simulink model "Modelisation_6_Validation_de_lineairisation_A_B_C"  (R2015a)
settings: Solver=ode45  StartTime=0.0  StopTime=0.2  MaxStep=0.0001  RelTol=1e-3
(part 1 of 2)
settings Model: Creator=user  LastModifiedBy=user

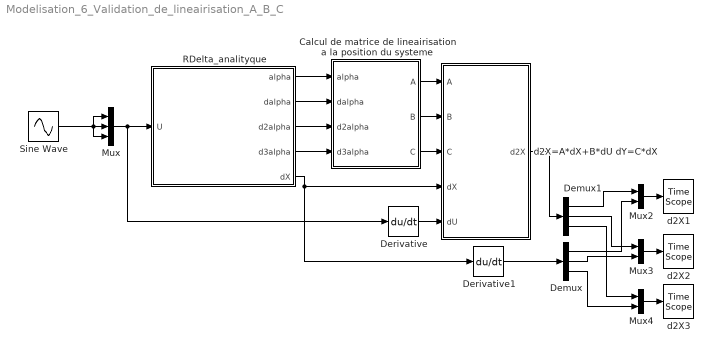
== system Modelisation_6_Validation_de_lineairisation_A_B_C ==
  Calcul de matrice de lineairisation a la position du systeme : Subsystem
  Demux : Demux  Outputs=3
  Demux1 : Demux  Outputs=3
  Derivative : Derivative
  Derivative1 : Derivative
  Mux : Mux  Inputs=3
  Mux2 : Mux  Inputs=2
  Mux3 : Mux  Inputs=2
  Mux4 : Mux  Inputs=2
  RDelta_analityque : Subsystem
      mask Display:
      | image(imread('DeltaImage2.PNG'))
      | port_label('input',1,'U')
      | port_label('output',1,'alpha')
      | port_label('output',2,'dalpha')
      | port_label('output',3,'d2alpha')
      | port_label('output',4,'d3alpha')
      | port_label('output',5,'dX')
  Sine Wave : Sin  Amplitude=0.5  SampleTime=0
  d2X1 : TimeScope  DefaultConfigurationName=spbscopes.TimeScopeBlockCfg
  d2X2 : TimeScope  DefaultConfigurationName=spbscopes.TimeScopeBlockCfg
  d2X3 : TimeScope  DefaultConfigurationName=spbscopes.TimeScopeBlockCfg
  d2X=A*dX+B*dU dY=C*dX : Subsystem
  wires:
  Calcul de matrice de lineairisation a la position du systeme/1(A) -> d2X=A*dX+B*dU dY=C*dX/1(A)
  Calcul de matrice de lineairisation a la position du systeme/2(B) -> d2X=A*dX+B*dU dY=C*dX/2(B)
  Calcul de matrice de lineairisation a la position du systeme/3(C) -> d2X=A*dX+B*dU dY=C*dX/3(C)
  RDelta_analityque/1(alpha) -> Calcul de matrice de lineairisation a la position du systeme/1(alpha)
  RDelta_analityque/2(dalpha) -> Calcul de matrice de lineairisation a la position du systeme/2(dalpha)
  RDelta_analityque/4(d3alpha) -> Calcul de matrice de lineairisation a la position du systeme/4(d3alpha)
  RDelta_analityque/3(d2alpha) -> Calcul de matrice de lineairisation a la position du systeme/3(d2alpha)
  RDelta_analityque/5(dX) -> d2X=A*dX+B*dU dY=C*dX/4(dX), Derivative1/1
  Derivative/1 -> d2X=A*dX+B*dU dY=C*dX/5(dU)
  Mux2/1 -> d2X1/1
  d2X=A*dX+B*dU dY=C*dX/1(d2X) -> Demux1/1
  Derivative1/1 -> Demux/1
  Demux1/1 -> Mux2/1
  Demux/1 -> Mux2/2
  Mux3/1 -> d2X2/1
  Demux1/2 -> Mux3/1
  Demux/2 -> Mux3/2
  Mux4/1 -> d2X3/1
  Demux1/3 -> Mux4/1
  Demux/3 -> Mux4/2
  Mux/1 -> Derivative/1, RDelta_analityque/1(U)
  Sine Wave/1 -> Mux/3, Mux/1, Mux/2

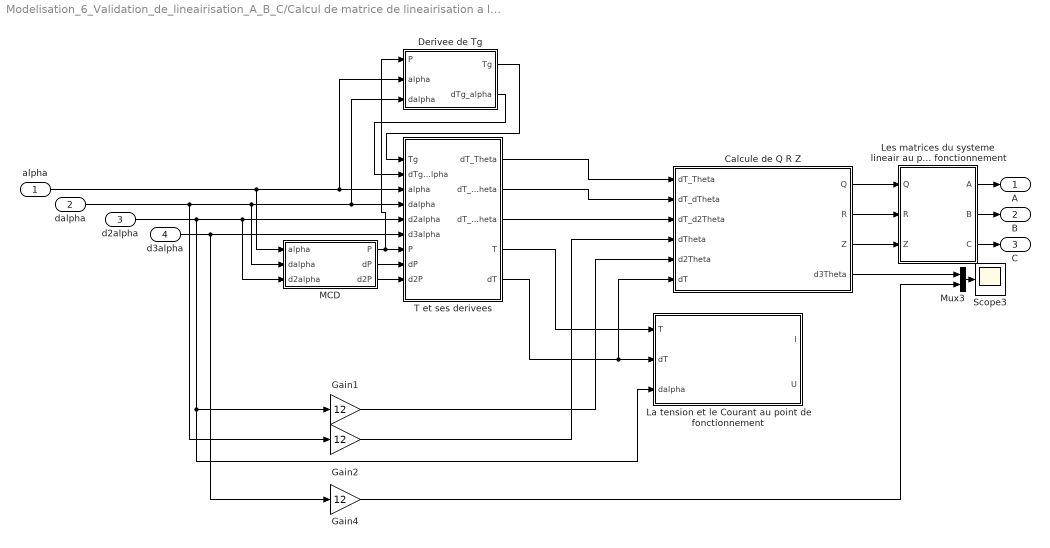
== system Modelisation_6_Validation_de_lineairisation_A_B_C/Calcul de matrice de lineairisation a la position du systeme ==
  alpha : Inport
  dalpha : Inport  Port=2
  d2alpha : Inport  Port=3
  d3alpha : Inport  Port=4
  "Calcule de Q R Z " : MATLAB Function  TreatAsAtomicUnit=on
  Derivee de Tg : Subsystem
  Gain1 : Gain  Gain=12
  Gain2 : Gain  Gain=12
  Gain4 : Gain  Gain=12
  La tension et le Courant au point de fonctionnement : MATLAB Function  TreatAsAtomicUnit=on
  Les matrices du systeme lineair au point de fonctionnement : MATLAB Function  TreatAsAtomicUnit=on
  MCD : MATLAB Function  TreatAsAtomicUnit=on
  Mux3 : Mux  Inputs=2
  Scope3 : Scope
      settings: TimeRange=2.077341948455237  YMin=-0.45  YMax=0.5
  T et ses derivees : Subsystem
  A : Outport
  B : Outport  Port=2
  C : Outport  Port=3
  wires:
  Les matrices du systeme lineair au point de fonctionnement/2(B) -> B/1
  Les matrices du systeme lineair au point de fonctionnement/3(C) -> C/1
  "Calcule de Q R Z "/1(Q) -> Les matrices du systeme lineair au point de fonctionnement/1(Q)
  "Calcule de Q R Z "/2(R) -> Les matrices du systeme lineair au point de fonctionnement/2(R)
  "Calcule de Q R Z "/3(Z) -> Les matrices du systeme lineair au point de fonctionnement/3(Z)
  Les matrices du systeme lineair au point de fonctionnement/1(A) -> A/1
  Gain4/1 -> Mux3/2
  "Calcule de Q R Z "/4(d3Theta) -> Mux3/1
  Mux3/1 -> Scope3/1
  Gain1/1 -> "Calcule de Q R Z "/5(d2Theta)
  Gain2/1 -> "Calcule de Q R Z "/4(dTheta)
  T et ses derivees/4(T) -> La tension et le Courant au point de fonctionnement/1(T)
  d3alpha/1 -> T et ses derivees/6(d3alpha), Gain4/1
  Derivee de Tg/1(Tg) -> T et ses derivees/1(Tg)
  Derivee de Tg/2(dTg_alpha) -> T et ses derivees/2(dTg_alpha)
  T et ses derivees/5(dT) -> La tension et le Courant au point de fonctionnement/2(dT), "Calcule de Q R Z "/6(dT)
  T et ses derivees/3(dT_d2Theta) -> "Calcule de Q R Z "/3(dT_d2Theta)
  T et ses derivees/2(dT_dTheta) -> "Calcule de Q R Z "/2(dT_dTheta)
  T et ses derivees/1(dT_Theta) -> "Calcule de Q R Z "/1(dT_Theta)
  d2alpha/1 -> MCD/3(d2alpha), T et ses derivees/5(d2alpha), La tension et le Courant au point de fonctionnement/3(dalpha), Gain1/1
  dalpha/1 -> MCD/2(dalpha), Derivee de Tg/3(dalpha), T et ses derivees/4(dalpha), Gain2/1
  alpha/1 -> MCD/1(alpha), T et ses derivees/3(alpha), Derivee de Tg/2(alpha)
  MCD/3(d2P) -> T et ses derivees/9(d2P)
  MCD/2(dP) -> T et ses derivees/8(dP)
  MCD/1(P) -> Derivee de Tg/1(P), T et ses derivees/7(P)

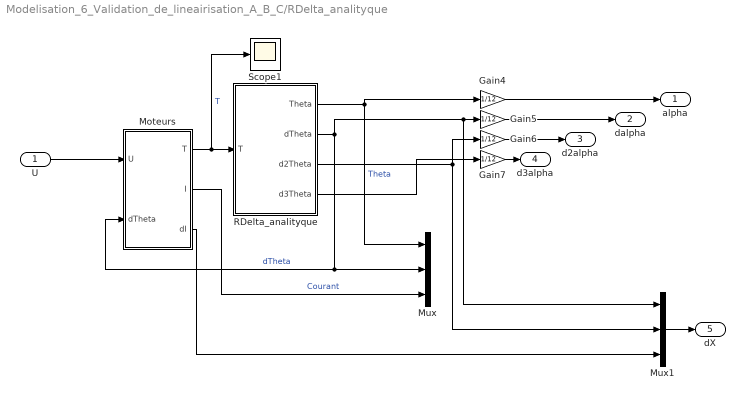
== system Modelisation_6_Validation_de_lineairisation_A_B_C/RDelta_analityque ==
  U : Inport
  Gain{4..7} (4 alike) : Gain  Gain=1/12
  Moteurs : Subsystem
  Mux : Mux  Inputs=3
  Mux1 : Mux  Inputs=3
  RDelta_analityque : Subsystem
  Scope1 : Scope
      settings: YMin=-0.013  YMax=-0.0095  SaveName=ScopeData3
  alpha : Outport
  dalpha : Outport  Port=2
  d2alpha : Outport  Port=3
  d3alpha : Outport  Port=4
  dX : Outport  Port=5
  wires:
  Moteurs/2(I) -> Mux/3  "Courant"
  U/1 -> Moteurs/1(U)
  RDelta_analityque/1(Theta) -> Mux/1, Gain4/1  "Theta"
  RDelta_analityque/2(dTheta) -> Moteurs/2(dTheta), Mux/2, Mux1/1, Gain5/1  "dTheta"
  Moteurs/1(T) -> Scope1/1, RDelta_analityque/1(T)  "T"
  RDelta_analityque/3(d2Theta) -> Mux1/2, Gain6/1
  RDelta_analityque/4(d3Theta) -> Gain7/1
  Mux1/1 -> dX/1
  Moteurs/3(dI) -> Mux1/3
  Gain4/1 -> alpha/1
  Gain5/1 -> dalpha/1
  Gain6/1 -> d2alpha/1
  Gain7/1 -> d3alpha/1

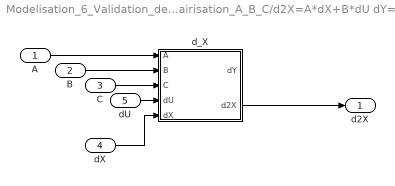
== system Modelisation_6_Validation_de_lineairisation_A_B_C/d2X=A*dX+B*dU dY=C*dX ==
  A : Inport
  B : Inport  Port=2
  C : Inport  Port=3
  dX : Inport  Port=4
  dU : Inport  Port=5
  d_X : MATLAB Function  TreatAsAtomicUnit=on
  d2X : Outport
  wires:
  B/1 -> d_X/2(B)
  C/1 -> d_X/3(C)
  A/1 -> d_X/1(A)
  dU/1 -> d_X/4(dU)
  dX/1 -> d_X/5(dX)
  d_X/2(d2X) -> d2X/1

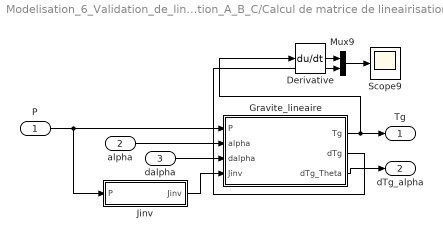
== system Modelisation_6_Validation_de_lineairisation_A_B_C/Calcul de matrice de lineairisation a la position du systeme/Derivee de Tg ==
  P : Inport
  alpha : Inport  Port=2
  dalpha : Inport  Port=3
  Derivative : Derivative
  Gravite_lineaire : MATLAB Function  TreatAsAtomicUnit=on
  Jinv : MATLAB Function  TreatAsAtomicUnit=on
  Mux9 : Mux  Inputs=2
  Scope9 : Scope
      settings: TimeRange=0.507510643892459  YMin=-1000  YMax=1000  SaveName=ScopeData12
  Tg : Outport
  dTg_alpha : Outport  Port=2
  wires:
  Gravite_lineaire/1(Tg) -> Derivative/1, Tg/1
  dalpha/1 -> Gravite_lineaire/3(dalpha)
  Gravite_lineaire/3(dTg_Theta) -> dTg_alpha/1
  Jinv/1(Jinv) -> Gravite_lineaire/4(Jinv)
  alpha/1 -> Gravite_lineaire/2(alpha)
  P/1 -> Gravite_lineaire/1(P), Jinv/1(P)
  Mux9/1 -> Scope9/1
  Derivative/1 -> Mux9/1
  Gravite_lineaire/2(dTg) -> Mux9/2

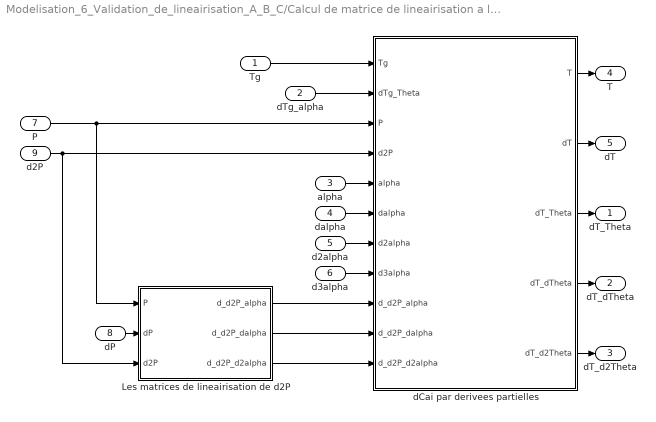
== system Modelisation_6_Validation_de_lineairisation_A_B_C/Calcul de matrice de lineairisation a la position du systeme/T et ses derivees ==
  Tg : Inport
  dTg_alpha : Inport  Port=2
  alpha : Inport  Port=3
  dalpha : Inport  Port=4
  d2alpha : Inport  Port=5
  d3alpha : Inport  Port=6
  P : Inport  Port=7
  dP : Inport  Port=8
  d2P : Inport  Port=9
  "Les matrices de lineairisation de d2P  " : MATLAB Function  TreatAsAtomicUnit=on
  "dCai par derivees partielles " : MATLAB Function  TreatAsAtomicUnit=on
  dT_Theta : Outport
  dT_dTheta : Outport  Port=2
  dT_d2Theta : Outport  Port=3
  T : Outport  Port=4
  dT : Outport  Port=5
  wires:
  "dCai par derivees partielles "/2(dT) -> dT/1
  "dCai par derivees partielles "/1(T) -> T/1
  d3alpha/1 -> "dCai par derivees partielles "/8(d3alpha)
  Tg/1 -> "dCai par derivees partielles "/1(Tg)
  dTg_alpha/1 -> "dCai par derivees partielles "/2(dTg_Theta)
  "dCai par derivees partielles "/5(dT_d2Theta) -> dT_d2Theta/1
  "dCai par derivees partielles "/4(dT_dTheta) -> dT_dTheta/1
  "dCai par derivees partielles "/3(dT_Theta) -> dT_Theta/1
  dP/1 -> "Les matrices de lineairisation de d2P  "/2(dP)
  d2alpha/1 -> "dCai par derivees partielles "/7(d2alpha)
  dalpha/1 -> "dCai par derivees partielles "/6(dalpha)
  alpha/1 -> "dCai par derivees partielles "/5(alpha)
  d2P/1 -> "dCai par derivees partielles "/4(d2P), "Les matrices de lineairisation de d2P  "/3(d2P)
  P/1 -> "dCai par derivees partielles "/3(P), "Les matrices de lineairisation de d2P  "/1(P)
  "Les matrices de lineairisation de d2P  "/1(d_d2P_alpha) -> "dCai par derivees partielles "/9(d_d2P_alpha)
  "Les matrices de lineairisation de d2P  "/3(d_d2P_d2alpha) -> "dCai par derivees partielles "/11(d_d2P_d2alpha)
  "Les matrices de lineairisation de d2P  "/2(d_d2P_dalpha) -> "dCai par derivees partielles "/10(d_d2P_dalpha)

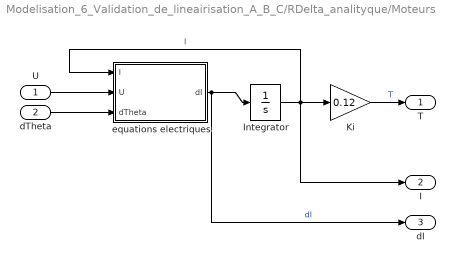
== system Modelisation_6_Validation_de_lineairisation_A_B_C/RDelta_analityque/Moteurs ==
  U : Inport
  dTheta : Inport  Port=2
  Integrator : Integrator  InitialCondition=-0.0108
  Ki : Gain  Gain=0.12
  equations electriques : MATLAB Function  TreatAsAtomicUnit=on
  T : Outport
  I : Outport  Port=2
  dI : Outport  Port=3
  wires:
  U/1 -> equations electriques/2(U)
  Integrator/1 -> Ki/1, I/1, equations electriques/1(I)  "I"
  equations electriques/1(dI) -> dI/1, Integrator/1  "dI"
  dTheta/1 -> equations electriques/3(dTheta)
  Ki/1 -> T/1  "T"

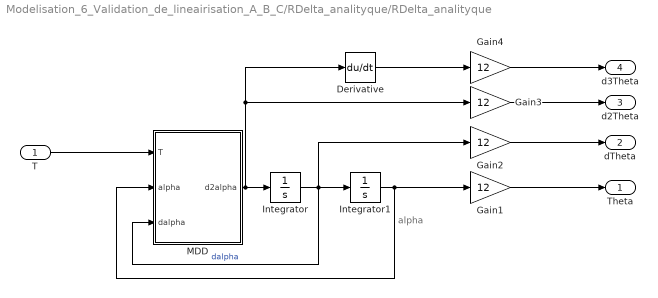
== system Modelisation_6_Validation_de_lineairisation_A_B_C/RDelta_analityque/RDelta_analityque ==
  note: alpha
  T : Inport
  Derivative : Derivative
  Gain{1..4} (4 alike) : Gain  Gain=12
  Integrator : Integrator  InitialCondition=[0;0;0]
  Integrator1 : Integrator  InitialCondition=0.0651*[1;1;1]
  MDD : Subsystem
  Theta : Outport
  dTheta : Outport  Port=2
  d2Theta : Outport  Port=3
  d3Theta : Outport  Port=4
  wires:
  MDD/1(d2alpha) -> Derivative/1, Gain3/1, Integrator/1
  Integrator/1 -> MDD/3(dalpha), Gain2/1, Integrator1/1  "dalpha"
  Integrator1/1 -> MDD/2(alpha), Gain1/1
  T/1 -> MDD/1(T)
  Gain1/1 -> Theta/1
  Gain2/1 -> dTheta/1
  Gain3/1 -> d2Theta/1
  Gain4/1 -> d3Theta/1
  Derivative/1 -> Gain4/1

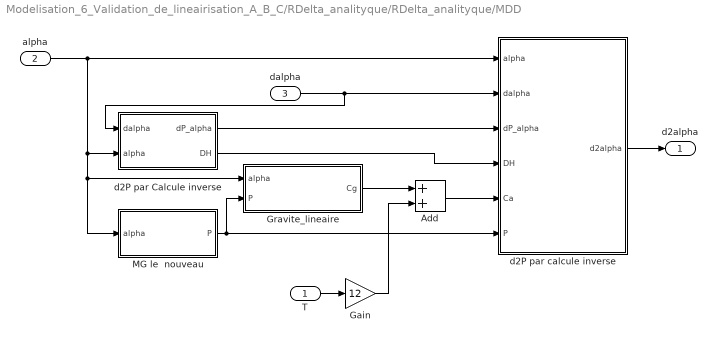
== system Modelisation_6_Validation_de_lineairisation_A_B_C/RDelta_analityque/RDelta_analityque/MDD ==
  T : Inport
  alpha : Inport  Port=2
  dalpha : Inport  Port=3
  Add : Sum
  Gain : Gain  Gain=12
  Gravite_lineaire : MATLAB Function  TreatAsAtomicUnit=on
  MG le  nouveau : MATLAB Function  TreatAsAtomicUnit=on
  "d2P par Calcule inverse " : Subsystem
  d2P par calcule inverse : MATLAB Function  TreatAsAtomicUnit=on
  d2alpha : Outport
  wires:
  d2P par calcule inverse/1(d2alpha) -> d2alpha/1
  "d2P par Calcule inverse "/1(dP_alpha) -> d2P par calcule inverse/3(dP_alpha)
  "d2P par Calcule inverse "/2(DH) -> d2P par calcule inverse/4(DH)
  MG le  nouveau/1(P) -> Gravite_lineaire/2(P), d2P par calcule inverse/6(P)
  Add/1 -> d2P par calcule inverse/5(Ca)
  Gravite_lineaire/1(Cg) -> Add/1
  dalpha/1 -> "d2P par Calcule inverse "/1(dalpha), d2P par calcule inverse/2(dalpha)
  alpha/1 -> MG le  nouveau/1(alpha), Gravite_lineaire/1(alpha), "d2P par Calcule inverse "/2(alpha), d2P par calcule inverse/1(alpha)
  T/1 -> Gain/1
  Gain/1 -> Add/2

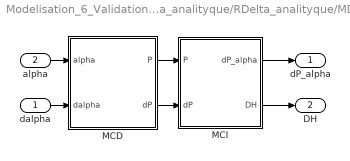
== system Modelisation_6_Validation_de_lineairisation_A_B_C/RDelta_analityque/RDelta_analityque/MDD/d2P par Calcule inverse  ==
  dalpha : Inport
  alpha : Inport  Port=2
  MCD : MATLAB Function  TreatAsAtomicUnit=on
  MCI : MATLAB Function  TreatAsAtomicUnit=on
  dP_alpha : Outport
  DH : Outport  Port=2
  wires:
  MCD/2(dP) -> MCI/2(dP)
  MCD/1(P) -> MCI/1(P)
  alpha/1 -> MCD/1(alpha)
  dalpha/1 -> MCD/2(dalpha)
  MCI/1(dP_alpha) -> dP_alpha/1
  MCI/2(DH) -> DH/1

== matlab function Modelisation_6_Validation_de_lineairisation_A_B_C/RDelta_analityque/RDelta_analityque/MDD/Gravite_lineaire ==
  data: alpha input; Cg output; P input
function Cg = fcn(alpha,P)

    alpha1=alpha(1) ;alpha2=alpha(2) ; alpha3=alpha(3) ;
    
%% les constantes:
l1 = 0.19992; 
l2 = 0.334; 
r = 0.126; 
phi2 = 2*pi/3;
phi3 = 4*pi/3;
A2=[cos(phi2) sin(phi2) 0 
     -sin(phi2) cos(phi2) 0
        0            0            1 ]; 
A3=[cos(phi3) sin(phi3) 0
     -sin(phi3) cos(phi3) 0
          0            0          1 ];
g = 9.98 ;
mBras = 0.083660682814532691 ;
mRoue =0.1805;
dBras = 0.058869490365843639 ;
dRoue = 0.0344586;
M2= 2*0.01438 ;
M3 = 0.0416;
shift = 0.0651;
%% Parametres :
    % A) les vecteurs OAi et OBi :
    OA1=[r ; 0 ; 0] ; OA2=[r*cos(phi2) ; r*sin(phi2) ; 0] ; OA3=[r*cos(phi3) ; r*sin(phi3) ; 0] ;
    OC1=[r+l1*cos(alpha1) ; 0 ; -l1*sin(alpha1) ]; 
    OC2=[(r+l1*cos(alpha2))*cos(phi2) ; (r+l1*cos(alpha2))*sin(phi2) ; -l1*sin(alpha2) ]; 
    OC3=[(r+l1*cos(alpha3))*cos(phi3) ; (r+l1*cos(alpha3))*sin(phi3) ; -l1*sin(alpha3) ]; 
    % B) Les vecteurs AiCi :
    A1C1=OC1-OA1 ; A2C2=OC2-OA2 ; A3C3=OC3-OA3 ;
    % Fin

%% ===============-------=====  Calcule de Cgi =====---------====================

% Les vecteurs unitaires portes par les bras paralleles : la nouvelle base
    u1=(P-OC1)/l2 ; u2=(P-OC2)/l2 ; u3=(P-OC3)/l2 ;
    U = [u1 u2 u3] ;

% Les forces aux points Ci ;
     N1=[-dBras*mBras*sin(shift) - dRoue*mRoue*cos(shift) ; 0 ; -dBras*mBras*cos(shift) + dRoue*mRoue*sin(shift)]*g/l1; 
    N2=[0 ;0 ; -M2*g/2] ;
    N=N1+N2;

% les effets totales appliquees a  la nacelle (N4):
    N4 = [0 ; 0 ; -(M3 + M2*3/2)*g] ;

% les composants de N4 sur les bras paralleles = Expression de N4 dans la Nouvelle base U:
    E1 = [1 0 0]; E2 = [0 1 0]; E3 = [0 0 1];
    Z = U\N4 ;
    Z1=(E1*Z)*u1; 
    Z2=(E2*Z)*u2;  
    Z3=(E3*Z)*u3 ;

% les matrices de transformation au plan OXiZi (Bi) :
    B1= [1 0 0; 0 0 0 ; 0 0 1] ;
    B2=B1*A2; B3=B1*A3 ;
% Le couple Cg1 au point de fonc P0:
Cg1 = E2*cross(A1C1,N + B1*Z1);
Cg2 = E2* cross(A2*A2C2,N + B2*Z2)  ;
Cg3 = E2* cross(A3*A3C3, N + B3*Z3) ;
Cg =[Cg1 ;Cg2;Cg3] ;

== matlab function Modelisation_6_Validation_de_lineairisation_A_B_C/Calcul de matrice de lineairisation a la position du systeme/MCD ==
  data: P output; alpha input; dalpha input; dP output; d2P output; d2alpha input
function [P,dP,d2P]= fcn(alpha,dalpha,d2alpha)

% alpha=alpha*pi/180;
% dalpha=dalpha*pi/180;
% d2alpha=d2alpha*pi/180;
alpha1=alpha(1) ;alpha2=alpha(2) ; alpha3=alpha(3) ;
dalpha1=dalpha(1) ;dalpha2=dalpha(2) ; dalpha3=dalpha(3) ;
d2alpha1=d2alpha(1) ;d2alpha2=d2alpha(2) ; d2alpha3=d2alpha(3) ;
%% Remarque: une letrre majiscule signifie un point ou un vecteur 
% tandit que un miniscule signifie la norme
%% les constantes
l1 = 0.19992; 
l2 = 0.334; 
r = 0.126; 
phi2 = 2*pi/3;
phi3 = 4*pi/3;
% Fin
%% les points Ci :
OC1=[r+l1*cos(alpha1) ; 0 ; -l1*sin(alpha1) ]; 
OC2=[(r+l1*cos(alpha2))*cos(phi2) ; (r+l1*cos(alpha2))*sin(phi2) ; -l1*sin(alpha2) ]; 
OC3=[(r+l1*cos(alpha3))*cos(phi3) ; (r+l1*cos(alpha3))*sin(phi3) ; -l1*sin(alpha3) ]; 
%% Les veccteurs CiCj :
C1C2=OC2-OC1; C2C3=OC3-OC2 ; C3C1=OC1-OC3;
%% vitesses de point Ci et CiCj:
% dC1= Q1*dAlpha1;
Q1=[-l1*sin(alpha1) ; 0 ; -l1*cos(alpha1)] ; 
Q2=[-l1*sin(alpha2)*cos(phi2) ; -l1*sin(alpha2)*sin(phi2) ; -l1*cos(alpha2)] ;
Q3=[-l1*sin(alpha3)*cos(phi3) ; -l1*sin(alpha3)*sin(phi3) ; -l1*cos(alpha3)] ;
dOC1=Q1*dalpha1 ;
dOC2=Q2*dalpha2 ;
dOC3=Q3*dalpha3 ;
dC1C2=dOC2-dOC1 ; dC2C3=dOC3-dOC2 ; dC3C1=dOC1-dOC3 ;

%% Les longueurs a,b,et c:
a=sqrt(C1C2'*C1C2);
b=sqrt(C2C3'*C2C3);
c=sqrt(C3C1'*C3C1);

%% Calcule de R et s :
p=a+b+c ; % le perimetre
p1=p-2*a ; p2=p-2*b ;  p3=p-2*c ; 
R=a*b*c/sqrt(p*p1*p2*p3); % le Rayon du C1C2C3
s=a*b*c/(2*R); % La surface
V1=C1C2/a; % les vecteures unitaires portes sur les segments
V2=C2C3/b;
V3=C3C1/c;
%% Calcule de n et w:
n=cross(C3C1,C1C2)/s ; % le Vecteur normale
w=sign(-a*a+c*c+b*b)*cross(n,V1) ;
%% les segments  tl=|TK| , ml=|ML| ,lp=|LP|
tl=sqrt(R^2-(a/2)^2);
ml=sqrt(R^2-(b/2)^2);
kl=sqrt(R^2-(c/2)^2);
lp=sqrt(l2^2-R^2) ;
%% les vitess de a,b,et c:
da=V1'*dC1C2;
db=V2'*dC2C3;
dc=V3'*dC3C1;
%% Calcule de dR:
dp=da+db+dc ;
dp1=dp-2*da ; dp2=dp-2*db ; dp3=dp-2*dc ;
dR = ( da/a + db/b + dc/c - 0.5*( dp/p + dp1/p1 + dp2/p2 + dp3/p3 ))*R ;
%dR = ( 1 - 4*R*tl/b/c)*R*da/a + (1-4*R*ml/a/c)*R*db/b + (1-4*R*kl/a/b)*R*dc/c ;
%% Calcule de :
dtl=(R*dR-a*da/4)/tl ;
dlp  = -R*dR/lp ;
ds = (da/a + db/b + dc/c - dR/R)*s ;
dV1=(dC1C2-da*V1)/a ;

dS = cross(dC3C1,C1C2) + cross(C3C1,dC1C2) ;
dn= (dS-ds*n)/s ;
dw=sign(-a*a+c*c+b*b)*(cross(dn,V1) + cross(n,dV1)) ;
% Calcule de P :
OL = (OC1+OC2)/2 + tl*w;
P = OL-lp*n ;
% Calcule de dP :
dOT = (dOC2 + dOC1)/2 ; 
dTL = dtl*w + tl*dw ;
dLP = -dlp*n - lp*dn ; 
dP = dOT + dTL + dLP ; 

%==================== d2OP en fonction de  d2alpha =======================
  %% L'acceleration de OCi  CiCj:
dQ1=[-l1*cos(alpha1) ; 0 ; l1*sin(alpha1)] ; dQ1t= dQ1*dalpha1 ;
dQ2=[-l1*cos(alpha2)*cos(phi2) ; -l1*cos(alpha2)*sin(phi2) ; l1*sin(alpha2)] ;dQ2t= dQ2*dalpha2 ;
dQ3=[-l1*cos(alpha3)*cos(phi3) ; -l1*cos(alpha3)*sin(phi3) ; l1*sin(alpha3)] ;dQ3t= dQ3*dalpha3 ;

d2C1 = dQ1*dalpha1^2 + Q1*d2alpha1;
d2C2 = dQ2*dalpha2^2 + Q2*d2alpha2;
d2C3 = dQ3*dalpha3^2 + Q3*d2alpha3;
d2C1C2=d2C2-d2C1 ;
d2C2C3=d2C3-d2C2 ; d2C3C1=d2C1-d2C3 ;
%% Les accelerations de a,b et c :
d2a = (d2C1C2'*C1C2 + dC1C2'*dC1C2 - da^2)/a ;
d2b = (d2C2C3'*C2C3 + dC2C3'*dC2C3 - db^2)/b ;
d2c = (d2C3C1'*C3C1 + dC3C1'*dC3C1 - dc^2)/c ;
%% L'acceleration de V1 :
d2V1=(d2C1C2 - 2*da*dV1 - d2a*V1)/a ;
%% L'acceleration de R :
d2p=d2a+d2b+d2c;
d2p1=d2p-2*d2a ; d2p2=d2p-2*d2b ; d2p3=d2p-2*d2c ;
d2R = ( d2a/a + d2b/b + d2c/c - 0.5*(d2p/p +  d2p1/p1 +  d2p2/p2 +  d2p3/p3 ) - (da/a)^2 -(db/b)^2 -(dc/c)^2 +0.5*( (dp/p)^2 +(dp1/p1)^2 +(dp2/p2)^2 +(dp3/p3)^2 ) +(dR/R)^2 )*R;
%% L'acceleration de S et s :
d2s = (d2a/a + d2b/b + d2c/c -d2R/R - (da/a)^2 -(db/b)^2 -(dc/c)^2 +(dR/R)^2 + (ds/s)^2)*s ;
d2S=cross(d2C3C1,C1C2) + 2*cross(dC3C1,dC1C2) + cross(C3C1,d2C1C2) ;
%% L'acceleraion de n et w ;
d2n=(d2S - d2s*n - 2*ds*dn)/s ;
d2w= sign(-a*a+c*c+b*b)*(cross(d2n,V1) +2*cross(dn,dV1) + cross(n,d2V1)) ;

%% Calcule de d2OT :
d2OT = (d2C1+d2C2)/2 ;
%% Calcule de d2TL ;
d2tl = (d2R*R + dR^2 - ( d2a*a + da^2 )/4 - dtl^2 )/tl ;
d2TL =d2tl*w + 2*dtl*dw + tl*d2w ;
%% Calcule de d2LP :
d2lp = -(d2R*R + dR^2 + dlp^2)/lp ;
d2LP = -d2lp*n -2*dlp*dn - lp*d2n ;
 
%% Calcule de d2P :
d2P = d2OT + d2TL + d2LP ;
% les commemtaires v=|V|

== matlab function Modelisation_6_Validation_de_lineairisation_A_B_C/d2X=A*dX+B*dU dY=C*dX/d_X ==
  data: dY output; A input; B input; C input; dU input; dX input; d2X output
function [dY,d2X]= fcn(A,B,C,dU,dX)

d2X= A*dX + B*dU ;
dY=C*dX ;

== matlab function Modelisation_6_Validation_de_lineairisation_A_B_C/RDelta_analityque/RDelta_analityque/MDD/MG le  nouveau ==
  data: alpha input; P output
function P =MGD(alpha)


alpha1=alpha(1) ;alpha2=alpha(2) ; alpha3=alpha(3) ;

%les constantes
l1 = 0.19992; 
l2 = 0.334; 
r = 0.126; 
phi2 = 2*pi/3;
phi3 = 4*pi/3;

%% Les points :
C1=[r+l1*cos(alpha1) ; 0 ; -l1*sin(alpha1) ]; 
C2=[(r+l1*cos(alpha2))*cos(phi2) ; (r+l1*cos(alpha2))*sin(phi2) ; -l1*sin(alpha2) ]; 
C3=[(r+l1*cos(alpha3))*cos(phi3) ; (r+l1*cos(alpha3))*sin(phi3) ; -l1*sin(alpha3) ]; 

%% Les vecteurs du triangle C1C2C3 et ses distances
C1C2= C2-C1 ; C2C3 =C3-C2 ; C3C1= C1-C3 ;
a=sqrt(C1C2'*C1C2) ; b=sqrt(C2C3'*C2C3)  ; c=sqrt(C3C1'*C3C1)  ;
 p= a+b+c ; % Le perimetre de C1C2C3
 R = a*b*c/sqrt(p*(p-2*a)*(p-2*b)*(p-2*c)) ;

 %% Calcule du point L 
 % Les vecteurs u et n:
 v1=C1C2/a ;
 n=cross(C3C1,C1C2)*2*R/(a*b*c) ;
 TL = sqrt(R^2-a^2/4) ;
 OL=(C1+C2)/2+TL*sign(-a*a+c*c+b*b)*cross(n,v1);
 %% Calcule du point E :
P=OL-sqrt(l2^2-R^2)*n ;

== matlab function Modelisation_6_Validation_de_lineairisation_A_B_C/RDelta_analityque/RDelta_analityque/MDD/d2P par Calcule inverse /MCD ==
  data: P output; alpha input; dalpha input; dP output
function [P,dP]= fcn(alpha,dalpha)

% alpha=alpha*pi/180;
% dalpha=dalpha*pi/180;
% d2alpha=d2alpha*pi/180;
alpha1=alpha(1) ;alpha2=alpha(2) ; alpha3=alpha(3) ;
dalpha1=dalpha(1) ;dalpha2=dalpha(2) ; dalpha3=dalpha(3) ;

%% Remarque: une letrre majiscule signifie un point ou un vecteur 
% tandit que un miniscule signifie la norme
%% les constantes
l1 = 0.19992; 
l2 = 0.334; 
r = 0.126; 
phi2 = 2*pi/3;
phi3 = 4*pi/3;
% Fin
%% les points Ci :
OC1=[r+l1*cos(alpha1) ; 0 ; -l1*sin(alpha1) ]; 
OC2=[(r+l1*cos(alpha2))*cos(phi2) ; (r+l1*cos(alpha2))*sin(phi2) ; -l1*sin(alpha2) ]; 
OC3=[(r+l1*cos(alpha3))*cos(phi3) ; (r+l1*cos(alpha3))*sin(phi3) ; -l1*sin(alpha3) ]; 
%% Les veccteurs CiCj :
C1C2=OC2-OC1; C2C3=OC3-OC2 ; C3C1=OC1-OC3;
%% vitesses de point Ci et CiCj:
% dC1= Q1*dAlpha1;
Q1=[-l1*sin(alpha1) ; 0 ; -l1*cos(alpha1)] ; 
Q2=[-l1*sin(alpha2)*cos(phi2) ; -l1*sin(alpha2)*sin(phi2) ; -l1*cos(alpha2)] ;
Q3=[-l1*sin(alpha3)*cos(phi3) ; -l1*sin(alpha3)*sin(phi3) ; -l1*cos(alpha3)] ;
dOC1=Q1*dalpha1 ;
dOC2=Q2*dalpha2 ;
dOC3=Q3*dalpha3 ;
dC1C2=dOC2-dOC1 ; dC2C3=dOC3-dOC2 ; dC3C1=dOC1-dOC3 ;

%% Les longueurs a,b,et c:
a=sqrt(C1C2'*C1C2);
b=sqrt(C2C3'*C2C3);
c=sqrt(C3C1'*C3C1);

%% Calcule de R et s :
p=a+b+c ; % le perimetre
p1=p-2*a ; p2=p-2*b ;  p3=p-2*c ; 
R=a*b*c/sqrt(p*p1*p2*p3); % le Rayon du C1C2C3
s=a*b*c/(2*R); % La surface
V1=C1C2/a; % les vecteures unitaires portes sur les segments
V2=C2C3/b;
V3=C3C1/c;
%% Calcule de n et w:
n=cross(C3C1,C1C2)/s ; % le Vecteur normale
w=sign(-a*a+c*c+b*b)*cross(n,V1) ;
%% les segments  tl=|TK| , ml=|ML| ,lp=|LP|
tl=sqrt(R^2-(a/2)^2);
ml=sqrt(R^2-(b/2)^2);
kl=sqrt(R^2-(c/2)^2);
lp=sqrt(l2^2-R^2) ;
%% les vitess de a,b,et c:
da=V1'*dC1C2;
db=V2'*dC2C3;
dc=V3'*dC3C1;
%% Calcule de dR:
dp=da+db+dc ;
dp1=dp-2*da ; dp2=dp-2*db ; dp3=dp-2*dc ;
dR = ( da/a + db/b + dc/c - 0.5*( dp/p + dp1/p1 + dp2/p2 + dp3/p3 ))*R ;
%dR = ( 1 - 4*R*tl/b/c)*R*da/a + (1-4*R*ml/a/c)*R*db/b + (1-4*R*kl/a/b)*R*dc/c ;
%% Calcule de :
dtl=(R*dR-a*da/4)/tl ;
dlp  = -R*dR/lp ;
ds = (da/a + db/b + dc/c - dR/R)*s ;
dV1=(dC1C2-da*V1)/a ;

dS = cross(dC3C1,C1C2) + cross(C3C1,dC1C2) ;
dn= (dS-ds*n)/s ;
dw=sign(-a*a+c*c+b*b)*(cross(dn,V1) + cross(n,dV1)) ;
% Calcule de P :
OL = (OC1+OC2)/2 + tl*w;
P = OL-lp*n ;
% Calcule de dP :
dOT = (dOC2 + dOC1)/2 ; 
dTL = dtl*w + tl*dw ;
dLP = -dlp*n - lp*dn ; 
dP = dOT + dTL + dLP ;

== matlab function Modelisation_6_Validation_de_lineairisation_A_B_C/RDelta_analityque/RDelta_analityque/MDD/d2P par Calcule inverse /MCI ==
  data: P input; dP input; dP_alpha output; DH output
    function [dP_alpha,DH]= fcn(P,dP)

    l1 = 0.19992; 
    l2 = 0.334; 
    r = 0.126; 
    phi2 = 2*pi/3;
    phi3 = 4*pi/3;

    %% Expression de P dans Ri
    % l'expression P1 dP1 et d2P1 ne se changent pas
    A2=[cos(phi2) sin(phi2) 0
        -sin(phi2) cos(phi2) 0
        0            0      1 ]; 
    A3=[cos(phi3) sin(phi3) 0
        -sin(phi3) cos(phi3) 0
        0            0      1 ];
     P2=A2*P; dP2=A2*dP; 
     P3=A3*P ; dP3=A3*dP ; 
        
    x1=P(1); y1=P(2) ; z1=P(3) ; 
    x2=P2(1); y2=P2(2) ; z2=P2(3) ;
    x3=P3(1); y3=P3(2) ; z3=P3(3) ;
   
    %% Parametres du Triangle AiCiBi :
    % Triangle 1 :
    AB1=sqrt(z1^2+(x1-r)^2);
    e1=sqrt(l2^2-y1^2); 
    AB2=sqrt(z2^2+(x2-r)^2);
    e2=sqrt(l2^2-y2^2);
    AB3=sqrt(z3^2+(x3-r)^2);
    e3=sqrt(l2^2-y3^2);

    %% calcul de alpha1
    beta1=atan2(-z1,x1-r);
    delta1=acos((AB1^2 + l1^2 - e1^2)/(2*l1*AB1));
    alpha1=beta1-delta1; 


    %% calcul de alpha2
    beta2=atan2(-z2,x2-r);
    delta2=acos((AB2^2 + l1^2 - e2^2)/(2*l1*AB2));
    alpha2=beta2-delta2; 


    %% calcul de alpha3
    beta3=atan2(-z3,x3-r);
    delta3=acos((AB3^2 + l1^2 - e3^2)/(2*l1*AB3));
    alpha3=beta3-delta3; 

% Tranformation au Deg
alpha=[alpha1;alpha2;alpha3]; % first solution


%% =================== Calcule de dalpha_i ====================================

% ---------------------------- Calcul de dAlpha1 ----------------------
% Calcule de dDelta1 :
BH1 = AB1-l1*cos(delta1);
D1=l1*AB1*sin(delta1) ;
dDelta1X = -BH1*(x1-r)/AB1/D1 ; 
dDelta1Y = -y1/D1 ; 
dDelta1Z = -BH1*z1/AB1/D1 ; 
Gdelta1=  [ dDelta1X , dDelta1Y , dDelta1Z] ;
dDelta1 = Gdelta1*dP ;
% Calcule de dBeta1 :
dBeta1Z=-(x1-r)/AB1^2 ; dBeta1X=z1/AB1^2 ;
Gbeta1=[ dBeta1X ,  0 , dBeta1Z] ;
dBeta1 = Gbeta1*dP;
% Calcule de dAlpha1 :
Galpha1=Gbeta1-Gdelta1 ;
dAlpha1 = Galpha1*dP ;

% ---------------------------- Calcul de dAlpha2 ----------------------
% Calcule de dDelta2 :
BH2 = AB2-l1*cos(delta2);
D2=l1*AB2*sin(delta2) ;
dDelta2X = -BH2*(x2-r)/AB2/D2 ; 
dDelta2Y = -y2/D2 ; 
dDelta2Z = -BH2*z2/AB2/D2 ; 
Gdelta2=  [ dDelta2X , dDelta2Y , dDelta2Z] ;
dDelta2 = Gdelta2*dP2 ;
% Calcule de dBeta2 :
dBeta2Z=-(x2-r)/AB2^2 ; dBeta2X=z2/AB2^2 ;
Gbeta2=[ dBeta2X ,  0 , dBeta2Z] ;
dBeta2 = Gbeta2*dP2;
% Calcule de dAlpha2 :
Galpha2=Gbeta2-Gdelta2 ;
dAlpha2 = Galpha2*dP2 ;

% ---------------------------- Calcul de dAlpha3 ----------------------
% Calcule de dDelta2 :
BH3 = AB3-l1*cos(delta3);
D3=l1*AB3*sin(delta3) ;
dDelta3X = -BH3*(x3-r)/AB3/D3 ; 
dDelta3Y = -y3/D3 ; 
dDelta3Z = -BH3*z3/AB3/D3 ; 
Gdelta3=  [ dDelta3X , dDelta3Y , dDelta3Z] ;
dDelta3 = Gdelta3*dP3 ;
% Calcule de dBeta3:
dBeta3Z=-(x3-r)/AB3^2 ; dBeta2X=z3/AB3^2 ;
Gbeta3=[ dBeta2X ,  0 , dBeta3Z] ;
dBeta3 = Gbeta3*dP3;
% Calcule de dAlpha3 :
Galpha3=Gbeta3-Gdelta3 ;
dAlpha3 = Galpha3*dP3 ;

dalpha=[ dAlpha1 ; dAlpha2 ; dAlpha3 ];

%% ===================== Calcule de d2alpha_i =================================
 
% ---------------------------- Calcul de d2Alpha1 ----------------------
% Calcule de d2Gama1 :
CH1=l1*sin(delta1);
AH1=l1*cos(delta1) ;
d2Delta1XX = -BH1*(x1-r)^2/(AB1^3*D1)*( AH1*e1^2/(BH1*CH1^2) + (AB1/(x1-r))^2 - 2 ) ;
d2Delta1YY = - (1+y1^2*AH1*AB1/D1^2 )  /D1;
d2Delta1ZZ  = -BH1*z1^2/(AB1^3*D1)*( AH1*e1^2/(BH1*CH1^2) + (AB1/z1)^2 -2 ) ;
d2Delta1XY = y1*(x1-r)*(CH1^2-AH1*BH1)/D1^3 ;
d2Delta1XZ = -BH1*(x1-r)*z1/(AB1^3*D1)*( AH1*e1^2/(BH1*CH1^2) - 2 ) ;
d2Delta1YZ = y1*z1*(CH1^2-AH1*BH1)/D1^3 ; 
Hdelta1=[ d2Delta1XX,d2Delta1XY,d2Delta1XZ ; d2Delta1XY, d2Delta1YY,d2Delta1YZ ;d2Delta1XZ , d2Delta1YZ,d2Delta1ZZ] ;

%Calcule de dBeta 1:
d2Beta1XX=-2*(x1-r)*z1/AB1^4 ; d2Beta1ZZ=-d2Beta1XX ; d2Beta1XZ = ((x1-r)^2-z1^2)/AB1^4 ;
Hbeta1= [d2Beta1XX , 0, d2Beta1XZ ; 0, 0, 0 ; d2Beta1XZ , 0 , d2Beta1ZZ ] ;

%Calcule de dAlpha1 :
Halpha1= Hbeta1 - Hdelta1; 


% ---------------------------- Calcul de d2Alpha2 ----------------------
% Calcule de d2Gama1 :
CH2=l1*sin(delta2);
AH2=l1*cos(delta2) ;
d2Delta2XX = -BH2*(x2-r)^2/(AB2^3*D2)*( AH2*e2^2/(BH2*CH2^2) + (AB2/(x2-r))^2 - 2 ) ;
d2Delta2YY = - (1+y2^2*AH2*AB2/D2^2 )  /D2;
d2Delta2ZZ  = -BH2*z2^2/(AB2^3*D2)*( AH2*e2^2/(BH2*CH2^2) + (AB2/z2)^2 -2 ) ;
d2Delta2XY = y2*(x2-r)*(CH2^2-AH2*BH2)/D2^3 ;
d2Delta2XZ = -BH2*(x2-r)*z2/(AB2^3*D2)*( AH2*e2^2/(BH2*CH2^2) - 2 ) ;
d2Delta2YZ = y2*z2*(CH2^2-AH2*BH2)/D2^3 ; 
Hdelta2=[ d2Delta2XX,d2Delta2XY,d2Delta2XZ ; d2Delta2XY, d2Delta2YY,d2Delta2YZ ;d2Delta2XZ , d2Delta2YZ,d2Delta2ZZ] ;

%Calcule de dBeta2:
d2Beta2XX=-2*(x2-r)*z2/AB2^4 ; d2Beta2ZZ=-d2Beta2XX ; d2Beta2XZ = ((x2-r)^2-z2^2)/AB2^4 ;
Hbeta2= [d2Beta2XX , 0, d2Beta2XZ ; 0, 0, 0 ; d2Beta2XZ , 0 , d2Beta2ZZ ] ;

%Calcule de dAlpha2 :
Halpha2= Hbeta2 - Hdelta2; 


% ---------------------------- Calcul de d2Alpha3 ----------------------
% Calcule de d2Gama3 :
CH3=l1*sin(delta3);
AH3=l1*cos(delta3) ;
d2Delta3XX = -BH3*(x3-r)^2/(AB3^3*D3)*( AH3*e3^2/(BH3*CH3^2) + (AB3/(x3-r))^2 - 2 ) ;
d2Delta3YY = - (1+y3^2*AH3*AB3/D3^2 )  /D3;
d2Delta3ZZ  = -BH3*z3^2/(AB3^3*D3)*( AH3*e3^2/(BH3*CH3^2) + (AB3/z3)^2 -2 ) ;
d2Delta3XY = y3*(x3-r)*(CH3^2-AH3*BH3)/D3^3 ;
d2Delta3XZ = -BH3*(x3-r)*z3/(AB3^3*D3)*( AH3*e3^2/(BH3*CH3^2) - 2 ) ;
d2Delta3YZ = y3*z3*(CH3^2-AH3*BH3)/D3^3 ; 
Hdelta3=[ d2Delta3XX,d2Delta3XY,d2Delta3XZ ; d2Delta3XY, d2Delta3YY,d2Delta3YZ ;d2Delta3XZ , d2Delta3YZ,d2Delta3ZZ] ;

%Calcule de dBeta3:
d2Beta3XX=-2*(x3-r)*z3/AB3^4 ; d2Beta3ZZ=-d2Beta3XX ; d2Beta3XZ = ((x3-r)^2-z3^2)/AB3^4 ;
Hbeta3= [d2Beta3XX , 0, d2Beta3XZ ; 0, 0, 0 ; d2Beta3XZ , 0 , d2Beta3ZZ ] ;

%Calcule de dAlpha3 :
Halpha3= Hbeta3 - Hdelta3; 


 % d2alpha=[d2Alpha1 ; d2Alpha2 ; d2Alpha3]; ou bien :

H = [dP'*Halpha1*dP ;dP2'*Halpha2*dP2 ;dP3'*Halpha3*dP3 ] ;
D = [Galpha1;Galpha2*A2;Galpha3*A3] ;
dP_alpha =eye(3)/D ;
DH = D\H ;
%% Clacule inverse de d2P :

% d2P =D\d2alpha-D\H ;

== matlab function Modelisation_6_Validation_de_lineairisation_A_B_C/RDelta_analityque/RDelta_analityque/MDD/d2P par calcule inverse ==
  data: alpha input; dalpha input; dP_alpha input; DH input; d2alpha output; Ca input; P input
function d2alpha  = fcn(alpha,dalpha, dP_alpha,DH,Ca,P)

alpha1=alpha(1) ;alpha2=alpha(2) ; alpha3=alpha(3) ;
dalpha1=dalpha(1) ;dalpha2=dalpha(2) ; dalpha3=dalpha(3) ;

%% les constantes
    l1 = 0.19992; 
    l2 = 0.334; 
    r = 0.126; 
    phi2 = 2*pi/3;
    phi3 = 4*pi/3;
A2=[cos(phi2) sin(phi2) 0
    -sin(phi2) cos(phi2) 0
    0            0      1 ]; 
A3=[cos(phi3) sin(phi3) 0
    -sin(phi3) cos(phi3) 0
    0            0      1 ];
% Constantes mecaniques
    J1=0.0071126;
    M2=2*0.01438  ;
    J2 = 2*0.00027499613;
    M3 = 0.04157 ;
    M4=2*J2/l2^2 ;
    
% Fin

% les vecteurs OAi et OCi :
OC1=[r+l1*cos(alpha1) ; 0 ; -l1*sin(alpha1) ]; 
OC2=[(r+l1*cos(alpha2))*cos(phi2) ; (r+l1*cos(alpha2))*sin(phi2) ; -l1*sin(alpha2) ]; 
OC3=[(r+l1*cos(alpha3))*cos(phi3) ; (r+l1*cos(alpha3))*sin(phi3) ; -l1*sin(alpha3) ]; 
%fin

% Les vecteurs unitaires portes par les bras paralleles : la nouvelle base
u1=(P-OC1)/l2 ; u2=(P-OC2)/l2 ; u3=(P-OC3)/l2 ;
%la matrice du transformation = La nouvelle base:
U = [u1 u2 u3] ;
%Uinv=inv(U);

%%  accelerations des points Ci :
% dOCi : la derivee partielle de OCi par rapport au alphai
% d2OCi : la deuxieme derivee partielle de OCi par rapport au alphai

dOC1_1=[-l1*sin(alpha1) ; 0 ; -l1*cos(alpha1)] ; 
dOC2_2=[-l1*sin(alpha2)*cos(phi2) ; -l1*sin(alpha2)*sin(phi2) ; -l1*cos(alpha2)] ;
dOC3_3=[-l1*sin(alpha3)*cos(phi3) ; -l1*sin(alpha3)*sin(phi3) ; -l1*cos(alpha3)] ;

d2OC1_1=[-l1*cos(alpha1) ; 0 ; l1*sin(alpha1)] ;
d2OC2_2=[-l1*cos(alpha2)*cos(phi2) ; -l1*cos(alpha2)*sin(phi2) ; l1*sin(alpha2)] ;
d2OC3_3=[-l1*cos(alpha3)*cos(phi3) ; -l1*cos(alpha3)*sin(phi3) ; l1*sin(alpha3)] ;

%Fin

%% ================ Le couple Cai en point de fonctionnement Couple1==================
% Parametres:
a1 = M2/4-M4/2 ; a2= M2/4 + M4/2; a3=M3 +3*a2 ; 
% la matrice de cross(AiCi,...)=aci  "ACi est exprimee dans le repere Ri"
ac1=[ 0 , l1*sin(alpha1) , 0 ; -l1*sin(alpha1) ,0 , -l1*cos(alpha1) ; 0 , l1*cos(alpha1),0]   ;
ac2=[ 0 , l1*sin(alpha2) , 0 ; -l1*sin(alpha2) ,0 , -l1*cos(alpha2) ; 0 , l1*cos(alpha2),0]   ;
ac3=[ 0 , l1*sin(alpha3) , 0 ; -l1*sin(alpha3) ,0 , -l1*cos(alpha3) ; 0 , l1*cos(alpha3),0]   ;
% Les matrices de projection
E1 = [1 0 0]; E2 = [0 1 0]; E3 = [0 0 1];
B1= [1 0 0; 0 0 0 ; 0 0 1] ; B2=B1*A2; B3=B1*A3 ;
%% 1)  Le couple Ca1 : 
G11=a3*(E2*ac1*B1*u1)*(E1/U) + a1*E2*ac1*B1 ;
G12=a1*(E2*ac1*B1*u1)*(E1/U)  ;
G13=a1*(E2*ac1*B1*u1)*(E1/U) + a2*E2*ac1*B1 ;
%Ca1=(J1+G13*dOC1_1)*d2alpha1+ G11*d2P +(G12*dOC2_2)*d2alpha2 + (G12*dOC3_3)*d2alpha3 +G13*d2OC1_1*dalpha1^2+ (G12*d2OC2_2)*dalpha2^2 + (G12*d2OC3_3)*dalpha3^2;
% Ca1 = J1*d2alpha1 + G11*d2P + G12* (d2OC2 +d2OC3) + G13*d2OC1 ;

%% 2)  Le couple Ca2 : 
G21=a3*(E2*ac2*B2*u2)*(E2/U) + a1*E2*ac2*B2 ;
G22=a1*(E2*ac2*B2*u2)*(E2/U)  ;
G23=a1*(E2*ac2*B2*u2)*(E2/U) + a2*E2*ac2*B2 ;
%Ca2=(J1+G23*dOC2_2)*d2alpha2+ G21*d2P +(G22*dOC1_1)*d2alpha1 + (G22*dOC3_3)*d2alpha3 +G23*d2OC2_2*dalpha2^2+ (G22*d2OC1_1)*dalpha1^2 + (G22*d2OC3_3)*dalpha3^2;
%Ca2 = J1*d2alpha2 + G21*d2P + G22* (d2OC1 +d2OC3) + G23*d2OC2 ;

%% 3)  Le couple Ca3 : 
G31=a3*(E2*ac3*B3*u3)*(E3/U) + a1*E2*ac3*B3 ;
G32=a1*(E2*ac3*B3*u3)*(E3/U)  ;
G33=a1*(E2*ac3*B3*u3)*(E3/U) + a2*E2*ac3*B3 ;
%Ca3=(J1+G33*dOC3_3)*d2alpha3+ G31*d2P +(G32*dOC2_2)*d2alpha2 + (G32*dOC1_1)*d2alpha1 + G33*d2OC3_3*dalpha3^2+ (G32*d2OC2_2)*dalpha2^2 + (G32*d2OC1_1)*dalpha1^2;
% Ca3 = J1*d2alpha3 + G31*d2P + G32* (d2OC2 +d2OC1) + G33*d2OC3 ;
% Fin

 %% ============= Calcule inverse de MDD (d2alpha en fonction de Ca ===========

e11= J1+G13*dOC1_1 ; 
e12 = (G12*dOC2_2) ;
e13 = (G12*dOC3_3) ;
b11 = G13*d2OC1_1 ;
b12 = (G12*d2OC2_2) ;
b13 =(G12*d2OC3_3) ;
% Ca1=e11*d2alpha1+e12*d2alpha2 + e13*d2alpha3 +b11*dalpha1^2+ b12*dalpha2^2 + b13*dalpha3^2 + G11*d2P ;

e21 = (G22*dOC1_1) ;
e22 = (J1+G23*dOC2_2) ;
e23 = (G22*dOC3_3) ;
b21 = (G22*d2OC1_1) ;
b22 = G23*d2OC2_2 ;
b23 = (G22*d2OC3_3) ;
% Ca2 = e22*d2alpha2 + e21*d2alpha1 + e23*d2alpha3 +b22*dalpha2^2 + b21*dalpha1^2 + b23*dalpha3^2 + G21*d2P ;

e31 = (G32*dOC1_1) ;
e32 =(G32*dOC2_2) ;
e33 =(J1+G33*dOC3_3);
b31 = (G32*d2OC1_1) ;
b32 =(G32*d2OC2_2) ;
b33 = G33*d2OC3_3 ;
% Ca3=e33*d2alpha3 +e32*d2alpha2 + e31*d2alpha1 + b33*dalpha3^2+ b32*dalpha2^2 + b31*dalpha1^2 + G31*d2P;

e=[e11 , e12 , e13 ; e21 , e22 , e23 ; e31 , e32 , e33] ;
b=[b11 , b12, b13 ; b21 , b22 , b23 ; b31, b32, b33] ;
G = [G11 ; G21 ; G31]  ;
dalphaCarre=[dalpha1^2 ; dalpha2^2; dalpha3^2] ;
% Ca = e*d2alpha + b*dalphaCarre + G*d2P ;
%% Calcule de d2alpha :

d2alpha =(e+G*dP_alpha)\(Ca - b*dalphaCarre + G*DH) ;

== matlab function Modelisation_6_Validation_de_lineairisation_A_B_C/Calcul de matrice de lineairisation a la position du systeme/Calcule de Q R Z  ==
  data: dT_Theta input; dT_dTheta input; dT_d2Theta input; Q output; R output; Z output; dTheta input; d2Theta input; dT input; d3Theta output
function [Q,R,Z,d3Theta]= fcn(dT_Theta,dT_dTheta,dT_d2Theta ,dTheta , d2Theta ,dT)

Z = eye(3,3)/ dT_d2Theta ;
Q= -Z*dT_Theta ;
R=-Z*dT_dTheta ;
d3Theta = Q*dTheta + R*d2Theta + Z*dT ;

== matlab function Modelisation_6_Validation_de_lineairisation_A_B_C/Calcul de matrice de lineairisation a la position du systeme/Derivee de Tg/Gravite_lineaire ==
  data: Tg output; dTg output; P input; alpha input; dalpha input; dTg_Theta output; Jinv input
function [Tg,dTg,dTg_Theta]= fcn(P,alpha,dalpha,Jinv)

    alpha1=alpha(1) ;alpha2=alpha(2) ; alpha3=alpha(3) ;
    
%% les constantes:
l1 = 0.19992; 
l2 = 0.334; 
r = 0.126; 
phi2 = 2*pi/3;
phi3 = 4*pi/3;
A2=[cos(phi2) sin(phi2) 0 
     -sin(phi2) cos(phi2) 0
        0            0            1 ]; 
A3=[cos(phi3) sin(phi3) 0
     -sin(phi3) cos(phi3) 0
          0            0          1 ];
g = 9.98 ;
mBras = 0.083660682814532691 ;
mRoue =0.1805;
dBras = 0.058869490365843639 ;
dRoue = 0.0344586;
M2= 2*0.01438 ;
M3 = 0.0416;
shift = 0.0651;
%% Parametres :
    % A) les vecteurs OAi et OBi :
    OA1=[r ; 0 ; 0] ; OA2=[r*cos(phi2) ; r*sin(phi2) ; 0] ; OA3=[r*cos(phi3) ; r*sin(phi3) ; 0] ;
    OC1=[r+l1*cos(alpha1) ; 0 ; -l1*sin(alpha1) ]; 
    OC2=[(r+l1*cos(alpha2))*cos(phi2) ; (r+l1*cos(alpha2))*sin(phi2) ; -l1*sin(alpha2) ]; 
    OC3=[(r+l1*cos(alpha3))*cos(phi3) ; (r+l1*cos(alpha3))*sin(phi3) ; -l1*sin(alpha3) ]; 
    % B) Les vecteurs AiCi :
    A1C1=OC1-OA1 ; A2C2=OC2-OA2 ; A3C3=OC3-OA3 ;
    % Fin

%% ===============-------=====  Calcule de Cgi =====---------====================

% Les vecteurs unitaires portes par les bras paralleles : la nouvelle base
    u1=(P-OC1)/l2 ; u2=(P-OC2)/l2 ; u3=(P-OC3)/l2 ;
    U = [u1 u2 u3] ;

% Les forces aux points Ci ;
     N1=[-dBras*mBras*sin(shift) - dRoue*mRoue*cos(shift) ; 0 ; -dBras*mBras*cos(shift) + dRoue*mRoue*sin(shift)]*g/l1; 
    N2=[0 ;0 ; -M2*g/2] ;
    N=N1+N2;

% les effets totales appliquees a  la nacelle (N4):
    N4 = [0 ; 0 ; -(M3 + M2*3/2)*g] ;

% les composants de N4 sur les bras paralleles = Expression de N4 dans la Nouvelle base U:
    E1 = [1 0 0]; E2 = [0 1 0]; E3 = [0 0 1];
    Z = U\N4 ;
    Z1=(E1*Z)*u1; 
    Z2=(E2*Z)*u2;  
    Z3=(E3*Z)*u3 ;

% les matrices de transformation au plan OXiZi (Bi) :
    B1= [1 0 0; 0 0 0 ; 0 0 1] ;
    B2=B1*A2; B3=B1*A3 ;
% Le couple Cg1 au point de fonc P0:
Cg1 = E2*cross(A1C1,N + B1*Z1);
Cg2 = E2* cross(A2*A2C2,N + B2*Z2)  ;
Cg3 = E2* cross(A3*A3C3, N + B3*Z3) ;
Cg =[Cg1 ;Cg2;Cg3] ;
Tg=Cg/12 ;
%% =========================== Linearisation ================================

% A) la derivee de ACi par rapport au alphai
    dAC1_1=[-l1*sin(alpha1) ; 0 ; -l1*cos(alpha1) ] ; 
    dAC2_2=A2'*[-l1*sin(alpha2); 0 ; -l1*cos(alpha2) ] ;
    dAC3_3=A3'*[-l1*sin(alpha3); 0 ; -l1*cos(alpha3)] ;

% B) les derivees partielles de la matrice U  par rapport au Apha_i
    % les derivees partielles de u1 par rapport au alphai
    du1_1=(Jinv*E1'-dAC1_1)/l2 ; 
    du1_2=(Jinv*E2')/l2 ; 
    du1_3=(Jinv*E3')/l2 ;
    % les derivees partielles de u2 par rapport au alphai
    du2_1=(Jinv*E1')/l2 ; 
    du2_2=(Jinv*E2'-dAC2_2)/l2 ; 
    du2_3=du1_3 ;
    % la derivee partielle de u3 par rapport au alphai
    du3_1=du2_1; 
    du3_2=du1_2; 
    du3_3=(Jinv*E3'-dAC3_3)/l2 ;
    % finalement
    dU_1=[du1_1 , du2_1 , du3_1]; % la derivee partielle de la matrice U par rapport au alpha1
    dU_2=[du1_2 , du2_2 , du3_2]; % la derivee partielle de la matrice U par rapport au alpha2
    dU_3=[du1_3 , du2_3 , du3_3]; % la derivee partielle de la matrice U par rapport au alpha3
    %dU = dU_1*dalpha(1) + dU_2*dalpha(2) +dU_3*dalpha(3) ;

% C) les derivees partielles de Z par rapport au alpha_i
    dZ_1=-U\dU_1*Z ;
    dZ_2=-U\dU_2*Z ;
    dZ_3=-U\dU_3*Z ;
    %dZ=dZ_1*Dalpha(1)+ dZ_2*Dalpha(2) + dZ_3*Dalpha(3) ;

% D) les derivee partilles de Zi par rapport au alpha_i :
    % La derivee de Z1 par rapport au alphai
    dZ1_1 = (E1*dZ_1)*u1+(E1*Z)*du1_1 ;
    dZ1_2 = (E1*dZ_2)*u1+(E1*Z)*du1_2 ;
    dZ1_3 = (E1*dZ_3)*u1+(E1*Z)*du1_3 ;
    % La derivee de Z2 par rapport au alphai
    dZ2_1 = (E2*dZ_1)*u2+(E2*Z)*du2_1 ;
    dZ2_2 = (E2*dZ_2)*u2+(E2*Z)*du2_2 ;
    dZ2_3 = (E2*dZ_3)*u2+(E2*Z)*du2_3 ;
    % La derivee de Z3 par rapport au alphai
    dZ3_1 = (E3*dZ_1)*u3+(E3*Z)*du3_1 ;
    dZ3_2 = (E3*dZ_2)*u3+(E3*Z)*du3_2 ;
    dZ3_3 = (E3*dZ_3)*u3+(E3*Z)*du3_3 ;
    %dZ3=dZ3_1*dalpha(1)+ dZ3_2*dalpha(2) + dZ3_3*dalpha(3) ;

%% E) les derivees partilles de Cgi par rapport au alpha_i :

    % 1) Les derivees partielles de Cg1:
    dCg1_1 = E2* cross(dAC1_1, N + B1*Z1) + E2*cross(A1C1 , B1*dZ1_1) ;
    dCg1_2 = E2*cross(A1C1 , B1*dZ1_2) ;
    dCg1_3 = E2*cross(A1C1 , B1*dZ1_3) ;
    dCg1_alpha = [dCg1_1 , dCg1_2 , dCg1_3] ; % dimension :1*3
    %dCg1= dCg1_1*Dalpha(1) + dCg1_2*Dalpha(2)  + dCg1_3*Dalpha(3) ;
    
    % 2) Les derivees partielles de Cg2:
    dCg2_1 = E2*cross(A2*A2C2 , B2*dZ2_1) ;
    dCg2_2 = E2* cross(A2*dAC2_2, N + B2*Z2) + E2*cross(A2*A2C2 , B2*dZ2_2) ;
    dCg2_3 = E2*cross(A2*A2C2 , B2*dZ2_3) ;
    dCg2_alpha = [dCg2_1 , dCg2_2 , dCg2_3] ;
    %dCg2= dCg2_1*Dalpha(1) + dCg2_2*Dalpha(2)  +dCg2_3*Dalpha(3) ;

    % 3) Les derivees partielles de Cg3:
    dCg3_1 = E2*cross(A3*A3C3 , B3*dZ3_1) ;
    dCg3_2 = E2*cross(A3*A3C3 , B3*dZ3_2) ;
    dCg3_3 = E2*cross(A3*dAC3_3, N + B3*Z3) + E2*cross(A3*A3C3 , B3*dZ3_3) ;
    dCg3_alpha = [dCg3_1 , dCg3_2 , dCg3_3] ;
    %dCg3= dCg3_1*Dalpha(1) + dCg3_2*Dalpha(2)  +dCg3_3*Dalpha(3) ;

dCg_alpha = [dCg1_alpha;dCg2_alpha;dCg3_alpha] ;

%% Les derivees partielles de Tg :
Theta = alpha*12 ; dTheta = dalpha*12 ; 
dTg_Theta = dCg_alpha/12^2 ; %% RQ :dTg_Theta = dTg_alpha/12

dTg = dTg_Theta * dTheta ;

== matlab function Modelisation_6_Validation_de_lineairisation_A_B_C/Calcul de matrice de lineairisation a la position du systeme/Derivee de Tg/Jinv ==
  data: P input; Jinv output
function Jinv= fcn(P)

l1 = 0.19992; 
l2 = 0.334; 
r = 0.126; 
phi2 = 2*pi/3;
phi3 = 4*pi/3;

%% projection de P sur Ri
A2=[cos(phi2) sin(phi2) 0
    -sin(phi2) cos(phi2) 0
    0            0      1 ]; 
A3=[cos(phi3) sin(phi3) 0
    -sin(phi3) cos(phi3) 0
    0            0      1 ];
P2=A2*P; P3=A3*P ;

x1=P(1); y1=P(2) ; z1=P(3) ; %% p1=p
x2=P2(1); y2=P2(2) ; z2=P2(3) ;
x3=P3(1); y3=P3(2) ; z3=P3(3) ;

%% Calcule de ABi et ei :
AB1=sqrt(z1^2+(x1-r)^2);
e1=sqrt(l2^2-y1^2); 
AB2=sqrt(z2^2+(x2-r)^2);
e2=sqrt(l2^2-y2^2);
AB3=sqrt(z3^2+(x3-r)^2);
e3=sqrt(l2^2-y3^2);

%% calcul de alpha1
gama1=acos((AB1^2 + l1^2 - e1^2)/(2*l1*AB1));
gama2=acos((AB2^2 + l1^2 - e2^2)/(2*l1*AB2));
gama3=acos((AB3^2 + l1^2 - e3^2)/(2*l1*AB3));

%% =========== Calcule de  J1  ================
% J1 est defini par : dalpha1= J1*dP
AB1 = sqrt(z1^2+(x1-r)^2);
AH1 = AB1-l1*cos(gama1);
D1=1/(l1*AB1*sin(gama1));
a1 = D1*AH1*(x1-r)/AB1 +  z1/( z1^2 + (x1-r)^2 );
a2 = D1*y1 ;
a3 = D1*AH1*z1/AB1 -(x1-r)/( z1^2 + (x1-r)^2 ) ;
j1= [a1 a2 a3] ;

%% =========== Calcule de  J2  ================
% J2 est defini par : dalpha2 = J2*A2*dP
AB2 = sqrt(z2^2+(x2-r)^2);
AH2 = AB2-l1*cos(gama2);
D2=1/(l1*AB2*sin(gama2));
a4 = D2*AH2*(x2-r)/AB2 + z2/( z2^2 + (x2-r)^2 ) ;
a5 = D2*y2;
a6 = D2*AH2*z2/AB2 -(x2-r)/( z2^2 + (x2-r)^2 );
j2=[a4 a5 a6]*A2;

%%  ========= (dAlpha3)  ================

AB3 = sqrt(z3^2+(x3-r)^2);
AH3 = AB3-l1*cos(gama3);
D3=1/(l1*AB3*sin(gama3));
a7 = D3*AH3*(x3-r)/AB3 + z3/( z3^2 + (x3-r)^2 );
a8 = D3*y3;
a9 = D3*AH3*z3/AB3 -(x3-r)/( z3^2 + (x3-r)^2 ) ;
j3=[ a7 a8 a9]*A3 ;

%% La matrice inverse de J
J=[ j1 ; j2 ; j3 ];
%  dAlpha=J*dp;   
Jinv=eye(3,3) /J;

== matlab function Modelisation_6_Validation_de_lineairisation_A_B_C/Calcul de matrice de lineairisation a la position du systeme/La tension et le Courant au point de fonctionnement ==
  data: T input; dT input; dalpha input; I output; U output
function [I,U]= fcn(T,dT,dalpha)

dTheta = dalpha*12 ;
b1=0.01 ; b2 = 0.005 ; b3 = 1 ; Ki=1 ;
I = T/Ki ;
dI = dT/Ki ;
U = (dI - b2*dTheta - b1*I)/b3 ;

== matlab function Modelisation_6_Validation_de_lineairisation_A_B_C/Calcul de matrice de lineairisation a la position du systeme/Les matrices du systeme lineair au point de fonctionnement ==
  data: Q input; A output; R input; Z input; B output; C output
function [A,B,C]= fcn(Q,R,Z)

%% Les matrices d'etat:
b1=0.01 ; b2 = 0.005 ; b3 = 1 ; Ki=0.12 ;

A= [  zeros(3,3)  , eye(3,3)   ,      zeros(3,3) 
           Q           ,    R         ,             Z*Ki    
     zeros(3,3), b2* eye(3,3)  , b1* eye(3,3)  ] ;
 B= [zeros(6,3) ; b3* eye(3,3)] ; 
 C= [eye(3,3), zeros(3,6)] ;

== matlab function Modelisation_6_Validation_de_lineairisation_A_B_C/RDelta_analityque/Moteurs/equations electriques ==
  data: I input; U input; dI output; dTheta input
function dI = fcn(I,U,dTheta)

b1=0.01 ; b2 = 0.005 ; b3 = 1 ; Ki=0.12 ;
 
dI = b2*dTheta + b1*I + b3*U ;
